simulink model "stateflow_naming_15b"  (R2015b)
settings: Solver=FixedStepDiscrete  StartTime=0.0  StopTime=10.0  RelTol=1e-3
PostLoadFcn:
  | % -------------------------------------------------------------------
  | %  Generated by MATLAB on 10-Feb-2017 13:23:05
  | %  MATLAB version: 9.1.0.441655 (R2016b)
  | % -------------------------------------------------------------------
  | 
  | 
  | diffName = Simulink.Signal;
  | diffName.CoderInfo.StorageClass = 'ExportedGlobal';
  | diffName.CoderInfo.Alias = '';
  | diffName.CoderInfo.Alignment = -1;
  | diffName.Description = '';
  | diffName.DataType = 'auto';
  | diffName.Min = [];
  | diffName.Max = [];
  | diffName.DocUnits = '';
  | diffName.Dimensions = -1;
  | diffName.DimensionsMode = 'auto';
  | diffName.Complexity = 'auto';
  | diffName.SampleTime = -1;
  | diffName.InitialValue = '';
  | 
  | myinput = Simulink.Signal;
  | myinput.CoderInfo.StorageClass = 'ExportedGlobal';
  | myinput.CoderInfo.Alias = '';
  | myinput.CoderInfo.Alignment = -1;
  | myinput.Description = '';
  | myinput.DataType = 'auto';
  | myinput.Min = [];
  | myinput.Max = [];
  | myinput.DocUnits = '';
  | myinput.Dimensions = -1;
  | myinput.DimensionsMode = 'auto';
  | myinput.Complexity = 'auto';
  | myinput.SampleTime = -1;
  | myinput.InitialValue = '';
  | 
  | out = Simulink.Signal;
  | out.CoderInfo.StorageClass = 'ExportedGlobal';
  | out.CoderInfo.Alias = '';
  | out.CoderInfo.Alignment = -1;
  | out.Description = '';
  | out.DataType = 'auto';
  | out.Min = [];
  | out.Max = [];
  | out.DocUnits = '';
  | out.Dimensions = -1;
  | out.DimensionsMode = 'auto';
  | out.Complexity = 'auto';
  | out.SampleTime = -1;
  | out.InitialValue = '';
  | 
  | out2 = Simulink.Signal;
  | out2.CoderInfo.StorageClass = 'ExportedGlobal';
  | out2.CoderInfo.Alias = '';
  | out2.CoderInfo.Alignment = -1;
  | out2.Description = '';
  | out2.DataType = 'auto';
  | out2.Min = [];
  | out2.Max = [];
  | out2.DocUnits = '';
  | out2.Dimensions = -1;
  | out2.DimensionsMode = 'auto';
  | out2.Complexity = 'auto';
  | out2.SampleTime = -1;
  | out2.InitialValue = '';
  | 
  | param = Simulink.Parameter;
  | param.Value = [1 2 3 4 5];
  | param.CoderInfo.StorageClass = 'ExportedGlobal';
  | param.CoderInfo.Alias = '';
  | param.CoderInfo.Alignment = -1;
  | param.Description = '';
  | param.DataType = 'auto';
  | param.Min = [];
  | param.Max = [];
  | param.DocUnits = '';
settings Model: Creator=amyyang  LastModifiedBy=amyyang
settings OptimizationCC: DefaultParameterBehavior=Inlined  OptimizeModelRefInitCode=on  LifeSpan=1
settings RTWCC: SystemTargetFile=ert.tlc  GenCodeOnly=on  TemplateMakefile=ert_default_tmf  Description=Embedded Coder  GenerateReport=on  IncludeHyperlinkInReport=on  LaunchReport=on  GenerateTraceInfo=on  GenerateTraceReport=on  GenerateTraceReportSl=on  GenerateTraceReportSf=on  GenerateTraceReportEml=on
settings CodeAppCC: IgnoreCustomStorageClasses=off
settings ERTTargetCC: GenerateSampleERTMain=on  InlinedParameterPlacement=NonHierarchical  ERTCustomFileTemplate=example_file_process.tlc
settings ConfigComp: CovModelRefEnable=Off

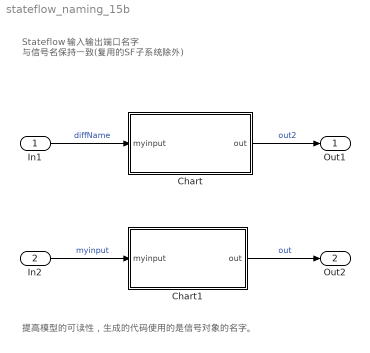
== system stateflow_naming_15b ==
  note: 提高模型的可读性，生成的代码使用的是信号对象的名字。
  note: Stateflow 输入输出端口名字
      | 与信号名保持一致(复用的SF子系统除外)
  In1 : Inport
  In2 : Inport  Port=2
  Chart : Stateflow chart  TreatAsAtomicUnit=on
  Chart1 : Stateflow chart  TreatAsAtomicUnit=on
  Out1 : Outport
  Out2 : Outport  Port=2
  wires:
  Chart/1(out) -> Out1/1  "out2"
  In1/1 -> Chart/1(myinput)  "diffName"
  Chart1/1(out) -> Out2/1  "out"
  In2/1 -> Chart1/1(myinput)  "myinput"

== stateflow chart stateflow_naming_15b/Chart1 ==
  (default) -> (junction 2) : {
      | out = param*myinput;
      | }
  data: out output; myinput input; param parameter

== stateflow chart stateflow_naming_15b/Chart ==
  (default) -> (junction 2) : {
      | out = param.*myinput;
      | }
  data: out output; myinput input; param parameter double size=5; data local
